simulink model "PIROSNavRec"  (Simulink 10.0)
settings: Solver=FixedStepAuto  StartTime=0.0  StopTime=inf  RelTol=1e-3
libraries: simulink x1, raspberrypilib x1, robotlib x1
settings Model: LogicAnalyzerSignalOrdering=05756065-db3f-4df3-b92b-4b7893301c68,af6bef99-8767-4027-895c-ece5892a47ed,0d8b97af-fcc9-4ae2-a994-46d894f70c73,71bc3483-cf3b-469d-958a-a2603a56a55f,03a37c5f-3e1c-4afb-9ce9-2a0d05751fd4,b07d944a-0d40-45b1-9495-e2296271bb99,bd67a88e-3c24-4961-9464-df372b02f3b7  Creator=earth  LastModifiedBy=earth
settings Model: SuppressorTable=|
  | <?xml version="1.0" encoding="UTF-8" standalone="yes" ?>
  | <!DOCTYPE boost_serialization>
  | <boost_serialization signature="serialization::archive" version="15">
  | <DiagnosticSuppressor class_id="0" tracking_level="0" version="6">
  | 	<Table class_id="1" tracking_level="0" version="0">
  | 		<count>1</count>
  | 		<bucket_count>2</bucket_count>
  | 		<item_version>0</item_version>
  | 		<item class_id="2" tracking_level="0" version="0">
  | 			<first class_id="3" tracking_level="0" version="6">
  | 				<Source class_id="4" tracking_level="0" version="0">
  | 					<count>1</count>
  | 					<item_version>0</item_version>
  | 					<item>PIROSNavRec/Counter Limited</item>
  | 				</Source>
  | 			</first>
  | 			<second class_id="5" tracking_level="0" version="6">
  | 				<SuppressedData class_id="6" tracking_level="0" version="0">
  | 					<count>2</count>
  | 					<bucket_count>5</bucket_count>
  | 					<item_version>0</item_version>
  | 					<item class_id="7" tracking_level="0" version="0">
  | 						<first class_id="8" tracking_level="0" version="6">
  | 							<ID>Simulink:DataType:WarningOverFlowDetected</ID>
  | 							<Cause>
  | 								<Source>
  | 									<count>0</count>
  | 									<item_version>0</item_version>
  | 								</Source>
  | 							</Cause>
  | 						</first>
  | 						<second class_id="9" tracking_level="0" version="6">
  | 							<Comment></Comment>
  | 							<User></User>
  | 							<LastModified class_id="10" tracking_level="0" version="0">
  | 								<ptime_date class_id="11" tracking_level="0" version="0">
  | 									<date>20160608</date>
  | 								</ptime_date>
  | 								<ptime_time_duration class_id="12" tracking_level="0" version="0">
  | 									<is_special>0</is_special>
  | 									<time_duration_hours>15</time_duration_hours>
  | 									<time_duration_minutes>23</time_duration_minutes>
  | 									<time_duration_seconds>17</time_duration_seconds>
  | 									<time_duration_fractional_seconds>0</time_duration_fractional_seconds>
  | 								</ptime_time_duration>
  | 							</LastModified>
  | 							<SuppressionType>1</SuppressionType>
  | 						</second>
  | 					</item>
  | 					<item>
  | 						<first>
  | 							<ID>SimulinkFixedPoint:util:Overflowoccurred</ID>
  | 							<Cause>
  | 								<Source>
  | 									<count>0</count>
  | 									<item_version>0</item_version>
  | 								</Source>
  | 							</Cause>
  | 						</first>
  | 						<second>
  | 							<Comment></Comment>
  | 							<User></User>
  | 							<LastModified>
  | 								<ptime_date>
  | 									<date>20160608</date>
  | 								</ptime_date>
  | 								<ptime_time_duration>
  | 									<is_special>0</is_special>
  | 									<time_duration_hours>15</time_duration_hours>
  | 									<time_duration_minutes>23</time_duration_minutes>
  | 									<time_duration_seconds>17</time_duration_seconds>
  | 									<time_duration_fractional_seconds>0</time_duration_fractional_seconds>
  | 								</ptime_time_duration>
  | 							</LastModified>
  | 							<SuppressionType>1</SuppressionType>
  | 						</second>
  | 					</item>
  | 				</SuppressedData>
  | 			</second>
  | 		</item>
  | 	</Table>
  | </DiagnosticSuppressor>
  | </boost_serialization>
settings DataIOCC: SaveFormat=Dataset  ReturnWorkspaceOutputs=on
settings OptimizationCC: EnhancedBackFolding=on  PassReuseOutputArgsAs=Individual arguments  ZeroExternalMemoryAtStartup=off  ZeroInternalMemoryAtStartup=off  LifeSpan=auto  MaxStackSize=64  OptimizeBlockOrder=speed  DifferentSizesBufferReuse=on  OptimizationCustomize=off  EfficientTunableParamExpr=on
settings DebuggingCC: UnderspecifiedInitializationDetection=Simplified  MergeDetectMultiDrivingBlocksExec=error  ParameterTunabilityLossMsg=error  SFUnexpectedBacktrackingDiag=error  SFNoUnconditionalDefaultTransitionDiag=error  SFExecutionAtInitializationDiag=warning  ArithmeticOperatorsInVariantConditions=error
settings HardwareCC: ProdLargestAtomicInteger=Long  ProdLargestAtomicFloat=Double  ProdIntDivRoundTo=Zero  ProdEndianess=LittleEndian  ProdHWDeviceType=ARM Compatible->ARM Cortex
settings ModelReferenceCC: PropagateSignalLabelsOutOfModel=on
settings SFSimCC: SimUseLocalCustomCode=on  MATLABDynamicMemAlloc=off  CustomCodeUndefinedFunction=FilterOut
settings RTWCC: Description=Embedded Coder  SystemTargetFile=ert.tlc  HardwareBoard=Robot Operating System (ROS)  TLCOptions="-aInlineSetEventsForThisBaseRateFcn=TLC_FALSE -aSuppressMultiTaskScheduler=TLC_FALSE  -aRateBasedStepFcn=0"  TemplateMakefile=ert_default_tmf  GenerateReport=on  RTWUseLocalCustomCode=on  Toolchain=Catkin  IncludeHyperlinkInReport=on  LaunchReport=on  TargetLang=C++  GenerateTraceInfo=on  GenerateTraceReport=on  GenerateTraceReportSl=on  GenerateTraceReportSf=on  GenerateTraceReportEml=on
settings MATStruct: className=codertarget.tools.BuildHook  argsTopModelOnly=[]  excludedModels=[]  includeReferencedModels=on  includeTopModel=on  enabled=on  UseCoderTarget=[1]  TargetHardware=Robot Operating System (ROS)  RTOS=Linux  RTOSBaseRateTaskPriority=40  DetectTaskOverruns=[0.0]  Scheduler_interrupt_source=[0.0]  DataVersion=2016.02  IPAddress=ros.codertarget.internal.DeviceParameters.getDeviceAddress  Port=17725  Verbose=[0]  RunInBackground=[1]  Configuration=TCP/IP  MaintainerName=ROS User  MaintainerEmail=rosuser@test.com  License=BSD  DeviceAddress=192.168.0.101  Username=ubuntu  BuildAction=None  Install=/opt/ros/melodic  CatkinWS=~/catkin_ws  ROSTimeStepping=0  ROSTimeNotification=0  StepNotify=/step_notify
settings CodeAppCC: ForceParamTrailComments=on  IgnoreCustomStorageClasses=off  OperatorAnnotations=on  SimulinkDataObjDesc=on  SFDataObjDesc=on  InsertBlockDesc=on  StateflowObjectComments=off
settings ConfigComp: CovMetricSettings=dwe  CovHtmlReporting=off  CovSaveCumulativeToWorkspaceVar=off  CovSaveSingleToWorkspaceVar=off

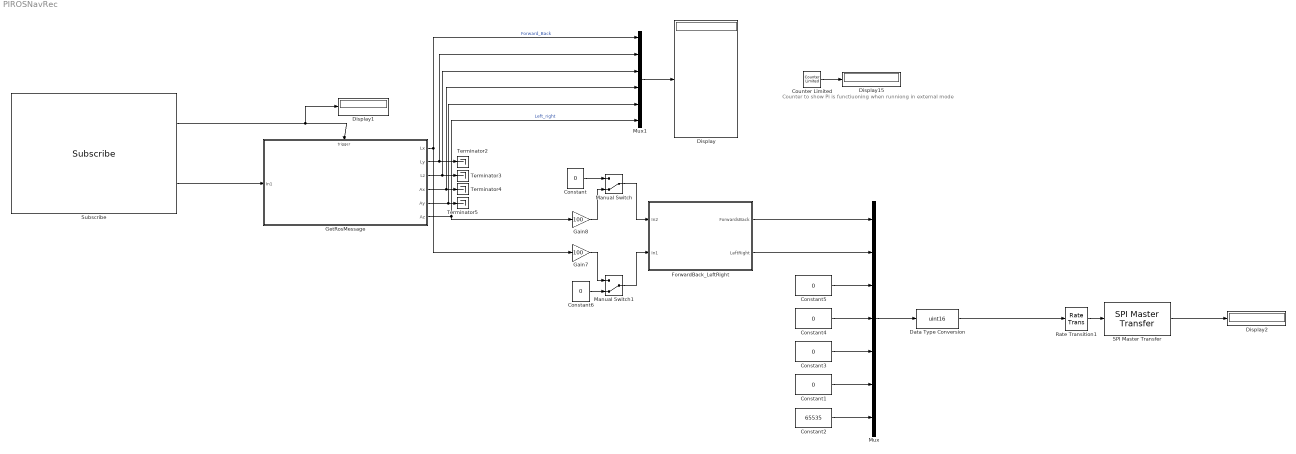
== system PIROSNavRec ==
  note: Counter to show Pi is functiuoning when runniong in external mode
  Constant{,1,3..6} (6 alike) : Constant  Value=0  OutDataTypeStr=single
  Constant2 : Constant  Value=65535  OutDataTypeStr=single
  Counter Limited : simulink/Sources/Counter Limited  uplimit=7  tsamp=1
  Data Type Conversion : DataTypeConversion  OutDataTypeStr=uint16  RndMeth=Round  SaturateOnIntegerOverflow=on
  Display{,1..2,15} (4 alike) : Display
      Display15 settings: Format=bank  Decimation=2
      Display2 settings: Format=bank  Decimation=2
  ForwardBack_LeftRight : Subsystem
  Gain7 : Gain  Gain=100
  Gain8 : Gain  Gain=100
  GetRosMessage : Subsystem
  Manual Switch : ManualSwitch  CurrentSetting=0
  Manual Switch1 : ManualSwitch  CurrentSetting=0
  Mux : Mux  Inputs=7
  Mux1 : Mux  Inputs=6
  Rate Transition1 : RateTransition  OutPortSampleTime=0.1
  SPI Master Transfer : raspberrypilib/SPI Master Transfer  BoardProperty=Pi 3 Model B+  SPIModule=uint32(0)  Mode=Master  BusSpeed=1000000  Pin=SPI0_CE0  FirstBitToTransfer=Most significant bit (MSB)  ClockMode=0  BlockFunction=Transfer  RegisterAddress=0  OutputDataType=int8  OutputDataLength=1
      settings: SourceProductName=Simulink Support Package for Raspberry Pi Hardware  SourceProductBaseCode=RASPPI
  Subscribe : robotlib/Subscribe  topicSource=Select from ROS network  topic=/planner/cmd_vel  messageType=geometry_msgs/Twist  sampleTime=0.1  messageQueueLength=1
      settings: SourceProductName=ROS Toolbox
  Terminator{2..5} (4 alike) : Terminator
  wires:
  GetRosMessage/4(Ax) -> Mux1/4, Terminator4/1
  Subscribe/1 -> Display1/1, GetRosMessage/Trigger
  GetRosMessage/3(Lz) -> Mux1/3, Terminator3/1
  GetRosMessage/2("Ly ") -> Mux1/2, Terminator2/1
  Mux1/1 -> Display/1
  GetRosMessage/5("Ay ") -> Mux1/5, Terminator5/1
  Subscribe/2 -> GetRosMessage/1(In1)
  GetRosMessage/1(Lx) -> Gain7/1, Mux1/1  "Forward_Back"
  Gain8/1 -> Manual Switch/2
  GetRosMessage/6("Az ") -> Mux1/6, Gain8/1  "Left_right"
  Gain7/1 -> Manual Switch1/1
  Constant2/1 -> Mux/7
  ForwardBack_LeftRight/2(LeftRight) -> Mux/2
  ForwardBack_LeftRight/1(ForwardsBack) -> Mux/1
  Constant1/1 -> Mux/6
  Constant3/1 -> Mux/5
  Constant4/1 -> Mux/4
  Constant5/1 -> Mux/3
  SPI Master Transfer/1 -> Display2/1
  Data Type Conversion/1 -> Rate Transition1/1
  Mux/1 -> Data Type Conversion/1
  Rate Transition1/1 -> SPI Master Transfer/1
  Counter Limited/1 -> Display15/1
  Constant/1 -> Manual Switch/1
  Manual Switch/1 -> ForwardBack_LeftRight/1(In2)
  Constant6/1 -> Manual Switch1/2
  Manual Switch1/1 -> ForwardBack_LeftRight/2(In1)

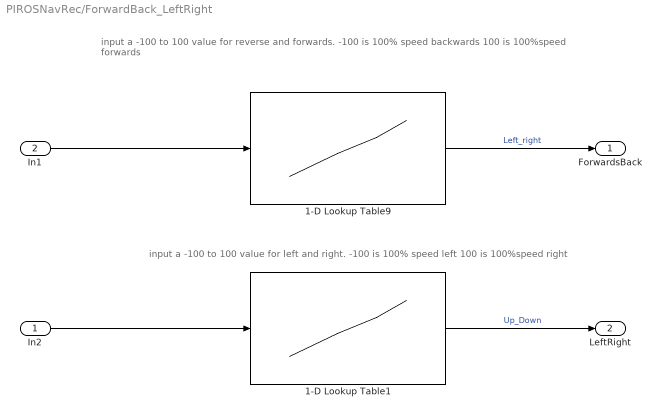
== system PIROSNavRec/ForwardBack_LeftRight ==
  note: input a -100 to 100 value for reverse and forwards. -100 is 100% speed backwards 100 is 100%speed forwards
  note: input a -100 to 100 value for left and right. -100 is 100% speed left 100 is 100%speed right
  In2 : Inport
  In1 : Inport  Port=2
  1-D Lookup Table1 : Lookup_n-D  NumberOfTableDimensions=1  BreakpointsForDimension1=[-100,-50,0,50,100]  BreakpointsForDimension1FirstPoint=0  BreakpointsForDimension1Spacing=1.8  Table=[2000;1750;1500;1250;1000]  ExtrapMethod=Clip  InternalRulePriority=Speed  RndMeth=Simplest  InputSameDT=on
  1-D Lookup Table9 : Lookup_n-D  NumberOfTableDimensions=1  BreakpointsForDimension1=[-100,-50,0,50,100]  BreakpointsForDimension1FirstPoint=0  BreakpointsForDimension1Spacing=1.8  Table=[1000;1250;1500;1750;2000]  ExtrapMethod=Clip  InternalRulePriority=Speed  RndMeth=Simplest  InputSameDT=on
  ForwardsBack : Outport
  LeftRight : Outport  Port=2
  wires:
  In1/1 -> 1-D Lookup Table9/1
  1-D Lookup Table1/1 -> LeftRight/1  "Up_Down"
  1-D Lookup Table9/1 -> ForwardsBack/1  "Left_right"
  In2/1 -> 1-D Lookup Table1/1

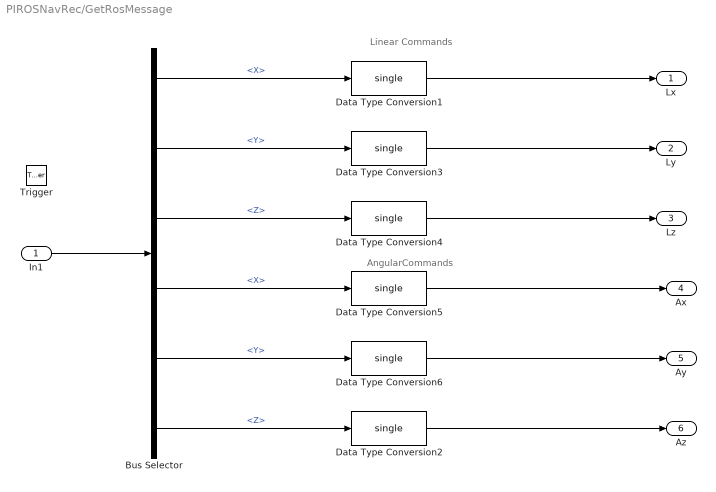
== system PIROSNavRec/GetRosMessage ==
  note: Linear Commands
  note: AngularCommands
  In1 : Inport
  Trigger : TriggerPort  VariantControl=Variant  PortDimensions=1
  Bus Selector : BusSelector  OutputSignals=Linear.X,Linear.Y,Linear.Z,Angular.X,Angular.Y,Angular.Z
  Data Type Conversion{1..6} (6 alike) : DataTypeConversion  OutDataTypeStr=single
  Lx : Outport  OutDataTypeStr=single
  "Ly " : Outport  Port=2
  Lz : Outport  Port=3
  Ax : Outport  Port=4
  "Ay " : Outport  Port=5
  "Az " : Outport  Port=6  OutDataTypeStr=single
  wires:
  Bus Selector/2 -> Data Type Conversion3/1  "<Y>"
  Bus Selector/1 -> Data Type Conversion1/1  "<X>"
  In1/1 -> Bus Selector/1
  Bus Selector/3 -> Data Type Conversion4/1  "<Z>"
  Bus Selector/4 -> Data Type Conversion5/1  "<X>"
  Bus Selector/5 -> Data Type Conversion6/1  "<Y>"
  Bus Selector/6 -> Data Type Conversion2/1  "<Z>"
  Data Type Conversion1/1 -> Lx/1
  Data Type Conversion2/1 -> "Az "/1
  Data Type Conversion3/1 -> "Ly "/1
  Data Type Conversion4/1 -> Lz/1
  Data Type Conversion5/1 -> Ax/1
  Data Type Conversion6/1 -> "Ay "/1
